simulink model "modelPOC"  (R2025b)
settings: Solver=FixedStepDiscrete  StartTime=0.0  StopTime=inf  FixedStep=1  RelTol=1e-3
model workspace (MAT data in the model file):
  gain = Simulink.Parameter
  gain.Value = 0
  gain.Complexity = 'real'
  gain.Dimensions = [1 1]
  gain.DataType = 'auto'
  k = Simulink.Parameter
  k.Value = 1
  k.Complexity = 'real'
  k.Dimensions = [1 1]
  k.DataType = 'auto'
values from neighbouring files (symbols this model uses):
  k = streamInd(m)    [soc_dvbs2_TxGeneration.m]
settings Model: Creator=KoayXianCong  LastModifiedBy=KoayXianCong
settings DataIOCC: LimitDataPoints=on
settings OptimizationCC: DefaultParameterBehavior=Inlined  EnhancedBackFolding=on  PassReuseOutputArgsAs=Individual arguments  ZeroExternalMemoryAtStartup=off  ZeroInternalMemoryAtStartup=off  OptimizeBlockOrder=speed  DifferentSizesBufferReuse=on  OptimizationCustomize=off  EfficientTunableParamExpr=on
settings DebuggingCC: ParameterTunabilityLossMsg=error
settings RTWCC: SystemTargetFile=ert.tlc  TemplateMakefile=ert_default_tmf  GenerateReport=on  LaunchReport=on  Description=Embedded Coder
settings CodeAppCC: ForceParamTrailComments=on  IgnoreCustomStorageClasses=off  OperatorAnnotations=on  SimulinkDataObjDesc=on  SFDataObjDesc=on  InsertBlockDesc=on
settings ERTTargetCC: ERTCustomFileTemplate=example_file_process.tlc  TargetLangStandard=C99 (ISO)  GenerateSampleERTMain=on

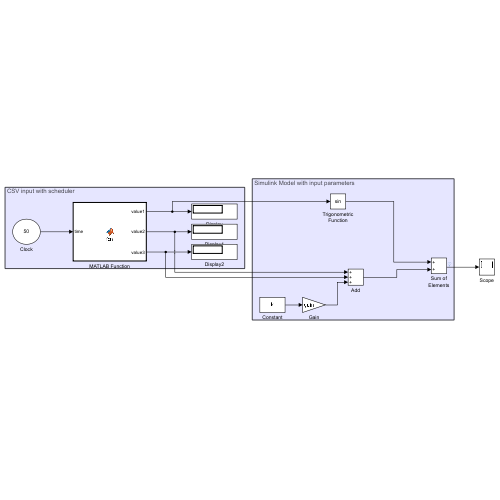
[thumbnail: Simulink's stored preview of the top-level diagram]
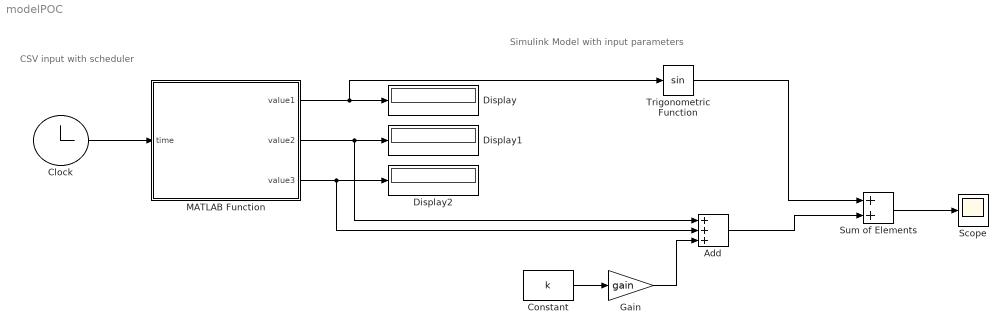
== system modelPOC ==
  note: Simulink Model with input parameters
  note: CSV input with scheduler
  Add : Sum  Inputs=+++
  Clock : Clock
  Constant : Constant  Value=k
  Display : Display
  Display1 : Display
  Display2 : Display
  Gain : Gain  Gain=gain
  MATLAB Function : MATLAB Function  TreatAsAtomicUnit=on
  Scope : Scope
      settings: ActiveDisplayYMinimum=-0.96670976283109966  ActiveDisplayYMaximum=8.7003878654798985
  Sum of Elements : Sum
  Trigonometric Function : Trigonometry
  wires:
  Clock/1 -> MATLAB Function/1(time)
  MATLAB Function/1(value1) -> Trigonometric Function/1, Display/1
  MATLAB Function/2(value2) -> Add/1, Display1/1
  MATLAB Function/3(value3) -> Display2/1, Add/2
  Constant/1 -> Gain/1
  Trigonometric Function/1 -> Sum of Elements/1
  Add/1 -> Sum of Elements/2
  Sum of Elements/1 -> Scope/1
  Gain/1 -> Add/3

== matlab function modelPOC/MATLAB Function ==
  data: value1 output; time input; value2 output; value3 output
function [value1, value2, value3] = fcn(time)
%#codegen

    persistent lastTime;
    persistent data;
    persistent errorCount;  % NEW: Track errors
    
    if isempty(lastTime)
        lastTime = 0;
        data = [0, 0, 0];
        errorCount = 0;  % NEW: Initialize error counter
    end
    
    % Change to 900 for 15 minutes (or keep 10 for testing)
    if time - lastTime >= 5  % CHANGED: 900 seconds = 15 minutes
        newData = readCSV();
        
        % NEW: Only update if valid data received
        if ~all(newData == 0)
            data = newData;
            errorCount = 0;
        else
            errorCount = errorCount + 1;
            % Keep using last good data if read fails
        end
        
        lastTime = time;
    end
    
    value1 = data(1);
    value2 = data(2);
    value3 = data(3);
end

function values = readCSV()
%#codegen
    values = [0.0, 0.0, 0.0];
    
    fid = fopen('input_data.csv', 'r');
    if fid == -1
        return;
    end
    
    line = fgets(fid);
    fclose(fid);  % Always close file
    
    if line == -1
        return;
    end
    
    % Simple manual parsing
    line = strtrim(line);
    
    % Find commas
    commaCount = 0;
    commaPos = zeros(1, 2);
    
    for i = 1:length(line)
        if line(i) == ','
            commaCount = commaCount + 1;
            if commaCount <= 2
                commaPos(commaCount) = i;
            end
        end
    end
    
    if commaCount >= 2
        % Extract strings
        str1 = line(1:commaPos(1)-1);
        str2 = line(commaPos(1)+1:commaPos(2)-1);
        str3 = line(commaPos(2)+1:end);
        
        % Convert using sscanf
        temp1 = sscanf(str1, '%f');
        temp2 = sscanf(str2, '%f');
        temp3 = sscanf(str3, '%f');
        
        if ~isempty(temp1)
            values(1) = temp1(1);
        end
        if ~isempty(temp2)
            values(2) = temp2(1);
        end
        if ~isempty(temp3)
            values(3) = temp3(1);
        end
    end
end
